simulink model "xNeuralSim_601"  (R2012b)
settings: Solver=FixedStepDiscrete  StartTime=0  StopTime=Inf  FixedStep=.0005  RelTol=1e-3
values from neighbouring files (symbols this model uses):
  cbhwlib_ver_major = 3    [buildXNeuralSim.m]    (also in xNeuralSim_Init.m)
  cbhwlib_ver_minor = 10    [buildXNeuralSim.m]    (also in xNeuralSim_Init.m = 9)
  enableNeuralSim = 1    [xNeuralSim_Init.m]
  max_num_cbpkts = 5    [xNeuralSim_Init.m]
  nch = 192    [xNeuralSim_Init.m]
  nsp_recv_port = 1001    [xNeuralSim_Init.m]
  nsp_send_port = 1002    [xNeuralSim_Init.m]
  sampleSendEnable_NSP1 = 1    [xNeuralSim_Init.m]
  sampleSendEnable_NSP2 = 1    [xNeuralSim_Init.m]
  spikeSendEnable_NSP1 = 1    [xNeuralSim_Init.m]
  spikeSendEnable_NSP2 = 1    [xNeuralSim_Init.m]
  unitMap = unitMap./repmat(sqrt(sum(unitMap.^2)), dimensions, 1)    [xNeuralSim_Init.m]
undefined symbols (not defined in the file or in its folder): macaddr
undefined symbols (not defined in the file): nsp1_pci_bus, nsp1_pci_slot
libraries: xpcethernetlib x15, xpcrtudplib x8, dspmtrx3 x7, xpclib x6, simulink x4, dspsrcs4 x2, xpciplib x2, xpcparallelportlib x1
(part 2 of 2)

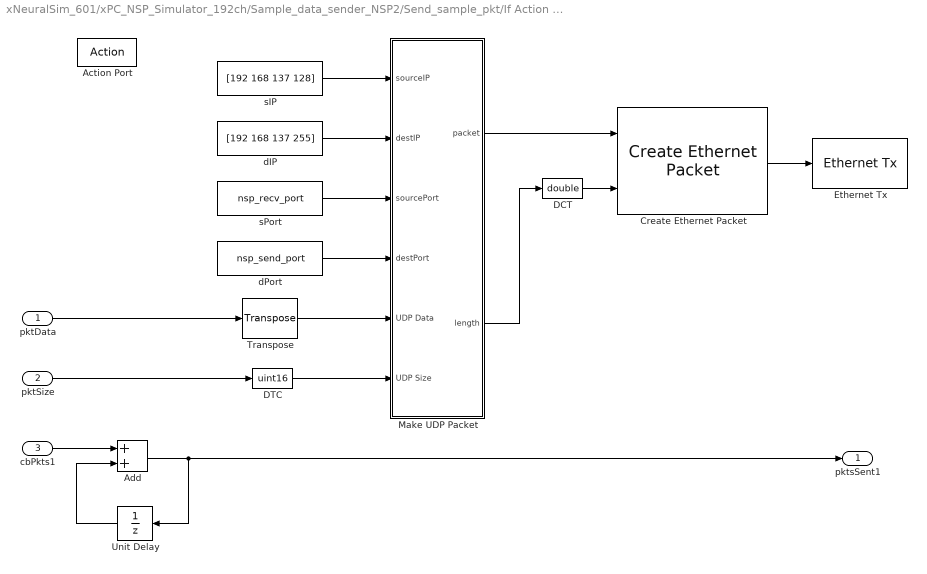
== system xNeuralSim_601/xPC_NSP_Simulator_192ch/Sample_data_sender_NSP2/Send_sample_pkt/If Action Subsystem ==
  pktData : Inport
  pktSize : Inport  Port=2
  cbPkts1 : Inport  Port=3
  Action Port : ActionPort  ActionType=then
  Add : Sum  AccumDataTypeStr=uint32  OutDataTypeStr=uint32
  Create Ethernet Packet : xpcethernetlib/Create Ethernet Packet   DstMac=macaddr('ff:ff:ff:ff:ff:ff')  EtherType=hex2dec('0800')
  DCT : DataTypeConversion  OutDataTypeStr=double
  DTC : DataTypeConversion  OutDataTypeStr=uint16
  Ethernet Tx : xpcethernetlib/Ethernet Tx   ID=2  SampleTime=-1
  Make UDP Packet : Subsystem
  Transpose : dspmtrx3/Transpose  Hermitian=off  overflowFlag=off
  Unit Delay : UnitDelay  SampleTime=-1
  dIP : Constant  Value=[192 168 137 255]  OutDataTypeStr=uint8
  dPort : Constant  Value=nsp_send_port  OutDataTypeStr=uint16
  sIP : Constant  Value=[192 168 137 128]  OutDataTypeStr=uint8
  sPort : Constant  Value=nsp_recv_port  OutDataTypeStr=uint16
  pktsSent1 : Outport  InitialOutput=0
  wires:
  Add/1 -> Unit Delay/1, pktsSent1/1
  Unit Delay/1 -> Add/2
  cbPkts1/1 -> Add/1
  DTC/1 -> Make UDP Packet/6(UDP Size)
  Make UDP Packet/2(length) -> DCT/1
  DCT/1 -> Create Ethernet Packet/2
  Make UDP Packet/1(packet) -> Create Ethernet Packet/1
  sPort/1 -> Make UDP Packet/3(sourcePort)
  Create Ethernet Packet/1 -> Ethernet Tx/1
  sIP/1 -> Make UDP Packet/1(sourceIP)
  dIP/1 -> Make UDP Packet/2(destIP)
  dPort/1 -> Make UDP Packet/4(destPort)
  Transpose/1 -> Make UDP Packet/5(UDP Data)
  pktData/1 -> Transpose/1
  pktSize/1 -> DTC/1

== system xNeuralSim_601/xPC_NSP_Simulator_192ch/Send_config_pkt/If Action Subsystem/Make UDP Packet ==
  note: UDP Data MUST be a uint8 vector of 1472 bytes
      | must pad data with 0s to reach 1472
  sourceIP : Inport
  destIP : Inport  Port=2
  sourcePort : Inport  Port=3
  destPort : Inport  Port=4
  UDP Data : Inport  Port=5
  UDP Size : Inport  Port=6
  Add IP Header : MATLAB Function  TreatAsAtomicUnit=on
  Add UDP Header : MATLAB Function  TreatAsAtomicUnit=on
  packet : Outport
  length : Outport  Port=2
  wires:
  UDP Size/1 -> Add UDP Header/6(UDP_size)
  Add IP Header/2(length) -> length/1
  Add IP Header/1(packet) -> packet/1
  UDP Data/1 -> Add UDP Header/5(UDP_data)
  destPort/1 -> Add UDP Header/4(destPort)
  sourcePort/1 -> Add UDP Header/3(sourcePort)
  destIP/1 -> Add IP Header/2(destIP), Add UDP Header/2(destIP)
  sourceIP/1 -> Add IP Header/1(sourceIP), Add UDP Header/1(sourceIP)
  Add UDP Header/1(packet) -> Add IP Header/3(IP_data)
  Add UDP Header/2(length) -> Add IP Header/4(IP_size)

== system xNeuralSim_601/xPC_NSP_Simulator_192ch/Send_heartbeat/If Action Subsystem/Make UDP Packet ==
  note: UDP Data MUST be a uint8 vector of 1472 bytes
      | must pad data with 0s to reach 1472
  sourceIP : Inport
  destIP : Inport  Port=2
  sourcePort : Inport  Port=3
  destPort : Inport  Port=4
  UDP Data : Inport  Port=5
  UDP Size : Inport  Port=6
  Add IP Header : MATLAB Function  TreatAsAtomicUnit=on
  Add UDP Header : MATLAB Function  TreatAsAtomicUnit=on
  packet : Outport
  length : Outport  Port=2
  wires:
  UDP Size/1 -> Add UDP Header/6(UDP_size)
  Add IP Header/2(length) -> length/1
  Add IP Header/1(packet) -> packet/1
  UDP Data/1 -> Add UDP Header/5(UDP_data)
  destPort/1 -> Add UDP Header/4(destPort)
  sourcePort/1 -> Add UDP Header/3(sourcePort)
  destIP/1 -> Add IP Header/2(destIP), Add UDP Header/2(destIP)
  sourceIP/1 -> Add IP Header/1(sourceIP), Add UDP Header/1(sourceIP)
  Add UDP Header/1(packet) -> Add IP Header/3(IP_data)
  Add UDP Header/2(length) -> Add IP Header/4(IP_size)

== system xNeuralSim_601/xPC_NSP_Simulator_192ch/Send_protocol_pkt/If Action Subsystem/Make UDP Packet ==
  note: UDP Data MUST be a uint8 vector of 1472 bytes
      | must pad data with 0s to reach 1472
  sourceIP : Inport
  destIP : Inport  Port=2
  sourcePort : Inport  Port=3
  destPort : Inport  Port=4
  UDP Data : Inport  Port=5
  UDP Size : Inport  Port=6
  Add IP Header : MATLAB Function  TreatAsAtomicUnit=on
  Add UDP Header : MATLAB Function  TreatAsAtomicUnit=on
  packet : Outport
  length : Outport  Port=2
  wires:
  UDP Size/1 -> Add UDP Header/6(UDP_size)
  Add IP Header/2(length) -> length/1
  Add IP Header/1(packet) -> packet/1
  UDP Data/1 -> Add UDP Header/5(UDP_data)
  destPort/1 -> Add UDP Header/4(destPort)
  sourcePort/1 -> Add UDP Header/3(sourcePort)
  destIP/1 -> Add IP Header/2(destIP), Add UDP Header/2(destIP)
  sourceIP/1 -> Add IP Header/1(sourceIP), Add UDP Header/1(sourceIP)
  Add UDP Header/1(packet) -> Add IP Header/3(IP_data)
  Add UDP Header/2(length) -> Add IP Header/4(IP_size)

== system xNeuralSim_601/xPC_NSP_Simulator_192ch/Send_response_pkt/If Action Subsystem/Make UDP Packet ==
  note: UDP Data MUST be a uint8 vector of 1472 bytes
      | must pad data with 0s to reach 1472
  sourceIP : Inport
  destIP : Inport  Port=2
  sourcePort : Inport  Port=3
  destPort : Inport  Port=4
  UDP Data : Inport  Port=5
  UDP Size : Inport  Port=6
  Add IP Header : MATLAB Function  TreatAsAtomicUnit=on
  Add UDP Header : MATLAB Function  TreatAsAtomicUnit=on
  packet : Outport
  length : Outport  Port=2
  wires:
  UDP Size/1 -> Add UDP Header/6(UDP_size)
  Add IP Header/2(length) -> length/1
  Add IP Header/1(packet) -> packet/1
  UDP Data/1 -> Add UDP Header/5(UDP_data)
  destPort/1 -> Add UDP Header/4(destPort)
  sourcePort/1 -> Add UDP Header/3(sourcePort)
  destIP/1 -> Add IP Header/2(destIP), Add UDP Header/2(destIP)
  sourceIP/1 -> Add IP Header/1(sourceIP), Add UDP Header/1(sourceIP)
  Add UDP Header/1(packet) -> Add IP Header/3(IP_data)
  Add UDP Header/2(length) -> Add IP Header/4(IP_size)

== system xNeuralSim_601/xPC_NSP_Simulator_192ch/Send_runlevel_pkt/If Action Subsystem/Make UDP Packet ==
  note: UDP Data MUST be a uint8 vector of 1472 bytes
      | must pad data with 0s to reach 1472
  sourceIP : Inport
  destIP : Inport  Port=2
  sourcePort : Inport  Port=3
  destPort : Inport  Port=4
  UDP Data : Inport  Port=5
  UDP Size : Inport  Port=6
  Add IP Header : MATLAB Function  TreatAsAtomicUnit=on
  Add UDP Header : MATLAB Function  TreatAsAtomicUnit=on
  packet : Outport
  length : Outport  Port=2
  wires:
  UDP Size/1 -> Add UDP Header/6(UDP_size)
  Add IP Header/2(length) -> length/1
  Add IP Header/1(packet) -> packet/1
  UDP Data/1 -> Add UDP Header/5(UDP_data)
  destPort/1 -> Add UDP Header/4(destPort)
  sourcePort/1 -> Add UDP Header/3(sourcePort)
  destIP/1 -> Add IP Header/2(destIP), Add UDP Header/2(destIP)
  sourceIP/1 -> Add IP Header/1(sourceIP), Add UDP Header/1(sourceIP)
  Add UDP Header/1(packet) -> Add IP Header/3(IP_data)
  Add UDP Header/2(length) -> Add IP Header/4(IP_size)

== system xNeuralSim_601/xPC_NSP_Simulator_192ch/Spike_data_sender_NSP1/Send_sample_pkt/If Action Subsystem ==
  pktData : Inport
  pktSize : Inport  Port=2
  cbPkts : Inport  Port=3
  Action Port : ActionPort  ActionType=then
  Add : Sum  AccumDataTypeStr=uint32  OutDataTypeStr=uint32
  Send_port_1002 : Subsystem  mask(send){Send1=192.168.137.255, Send2=nsp_send_port, Send3=nsp_recv_port, Send4=-1}
      mask prompts: Send1 "IP address to send to (255.255.255.255 for broadcast):"; Send2 "Remote IP port to send to:"; Send3 "Use the following local IP port (-1 for automatic assignment):"; Send4 "Sample time:"
      mask init:
      | Send1 = ipaddr(Send1);
      mask Help: helpview(fullfile(docroot, 'mapfiles', 'xpc.map'), 'RT_UDP_SEND')
      mask Display: disp('UDP\nSend')
  Unit Delay : UnitDelay  SampleTime=-1
  pktsSent : Outport  InitialOutput=0
  wires:
  Add/1 -> Unit Delay/1, pktsSent/1
  Unit Delay/1 -> Add/2
  cbPkts/1 -> Add/1
  pktData/1 -> Send_port_1002/1(In1)
  pktSize/1 -> Send_port_1002/2(In2)

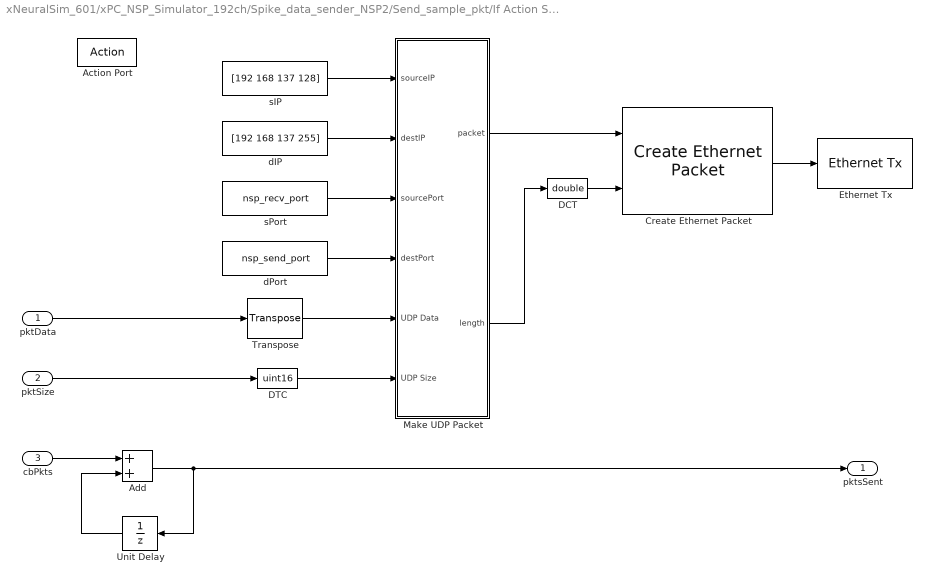
== system xNeuralSim_601/xPC_NSP_Simulator_192ch/Spike_data_sender_NSP2/Send_sample_pkt/If Action Subsystem ==
  pktData : Inport
  pktSize : Inport  Port=2
  cbPkts : Inport  Port=3
  Action Port : ActionPort  ActionType=then
  Add : Sum  AccumDataTypeStr=uint32  OutDataTypeStr=uint32
  Create Ethernet Packet : xpcethernetlib/Create Ethernet Packet   DstMac=macaddr('ff:ff:ff:ff:ff:ff')  EtherType=hex2dec('0800')
  DCT : DataTypeConversion  OutDataTypeStr=double
  DTC : DataTypeConversion  OutDataTypeStr=uint16
  Ethernet Tx : xpcethernetlib/Ethernet Tx   ID=2  SampleTime=-1
  Make UDP Packet : Subsystem
  Transpose : dspmtrx3/Transpose  Hermitian=off  overflowFlag=off
  Unit Delay : UnitDelay  SampleTime=-1
  dIP : Constant  Value=[192 168 137 255]  OutDataTypeStr=uint8
  dPort : Constant  Value=nsp_send_port  OutDataTypeStr=uint16
  sIP : Constant  Value=[192 168 137 128]  OutDataTypeStr=uint8
  sPort : Constant  Value=nsp_recv_port  OutDataTypeStr=uint16
  pktsSent : Outport  InitialOutput=0
  wires:
  Add/1 -> Unit Delay/1, pktsSent/1
  Unit Delay/1 -> Add/2
  cbPkts/1 -> Add/1
  DTC/1 -> Make UDP Packet/6(UDP Size)
  Make UDP Packet/2(length) -> DCT/1
  DCT/1 -> Create Ethernet Packet/2
  Make UDP Packet/1(packet) -> Create Ethernet Packet/1
  sPort/1 -> Make UDP Packet/3(sourcePort)
  Create Ethernet Packet/1 -> Ethernet Tx/1
  sIP/1 -> Make UDP Packet/1(sourceIP)
  dIP/1 -> Make UDP Packet/2(destIP)
  dPort/1 -> Make UDP Packet/4(destPort)
  Transpose/1 -> Make UDP Packet/5(UDP Data)
  pktData/1 -> Transpose/1
  pktSize/1 -> DTC/1

== system xNeuralSim_601/xPC_NSP_Simulator_192ch/Sample_data_sender_NSP1/Send_sample_pkt/If Action Subsystem/Send_port_1002 ==
  In1 : Inport  OutDataTypeStr=uint8
  In2 : Inport  Port=2  OutDataTypeStr=double
  "Compose " : S-Function  FunctionName=xpcnbcompose  EnableBusSupport=off  mask(xpcnbcompose){}
      mask help: Network Buffer Compose
      mask init:
      | mxpcnbcompose(2);
      mask Help: helpview(fullfile(docroot, 'mapfiles', 'xpc.map'), 'NB_Compose')
      mask Display: disp('NB Compose\n');port_label('input', 2, 'length');
  "UDP Produce " : S-Function  Priority=5  FunctionName=xpcudpproduce  Parameters=Group, SrcIp, sip, DstIp, dip, LocPort, lup, RemPort, rup, SampleTime  EnableBusSupport=off  mask(udpproduce){Group=0, sip=Auto, SrcIp=0.0.0.0, dip=Specify, DstIp=Send1, rup=Specify, RemPort=Send2, lup=Auto, LocPort=Send3, SampleTime=Send4}
      mask prompts: Group "IP Group"; sip "Source IP Address"; SrcIp "Source IP Address"; dip "Destination IP Address"; DstIp "IP address to send to (255.255.255.255 for broadcast):"; rup "Remote UDP Port"; RemPort "Remote IP port to send to:"; lup "Local UDP Port"; LocPort "Use the following local IP port (-1 for automatic assignment):"; SampleTime "Sample time:"
      mask help: UDP Produce
      mask init:
      | if LocPort == -1
      |     lup = 3;
      | else
      |     lup = 1;
      | end
      | 
      | SrcIp = ipaddr(SrcIp);
      | DstIp = ipaddr(DstIp);
      mask Help: helpview(fullfile(docroot, 'mapfiles', 'xpc.map'), 'RT_UDP_PRODUCE')
      mask TypeOptions sip: Specify | Port | Auto
      mask TypeOptions dip: Specify | Port
      mask TypeOptions rup: Specify | Port
      mask TypeOptions lup: Specify | Port | Auto
      mask Display: disp('UDP Produce');
  "UDP Tx " : xpciplib/UDP Tx   Priority=5  Group=0  TTL=-1  ToS=-1  SampleTime=Send4
  wires:
  "UDP Produce "/1 -> "UDP Tx "/1
  "Compose "/1 -> "UDP Produce "/1
  In1/1 -> "Compose "/1
  In2/1 -> "Compose "/2

== system xNeuralSim_601/xPC_NSP_Simulator_192ch/Sample_data_sender_NSP2/Send_sample_pkt/If Action Subsystem/Make UDP Packet ==
  note: UDP Data MUST be a uint8 vector of 1472 bytes
      | must pad data with 0s to reach 1472
  sourceIP : Inport
  destIP : Inport  Port=2
  sourcePort : Inport  Port=3
  destPort : Inport  Port=4
  UDP Data : Inport  Port=5
  UDP Size : Inport  Port=6
  Add IP Header : MATLAB Function  TreatAsAtomicUnit=on
  Add UDP Header : MATLAB Function  TreatAsAtomicUnit=on
  packet : Outport
  length : Outport  Port=2
  wires:
  UDP Size/1 -> Add UDP Header/6(UDP_size)
  Add IP Header/2(length) -> length/1
  Add IP Header/1(packet) -> packet/1
  UDP Data/1 -> Add UDP Header/5(UDP_data)
  destPort/1 -> Add UDP Header/4(destPort)
  sourcePort/1 -> Add UDP Header/3(sourcePort)
  destIP/1 -> Add IP Header/2(destIP), Add UDP Header/2(destIP)
  sourceIP/1 -> Add IP Header/1(sourceIP), Add UDP Header/1(sourceIP)
  Add UDP Header/1(packet) -> Add IP Header/3(IP_data)
  Add UDP Header/2(length) -> Add IP Header/4(IP_size)

== system xNeuralSim_601/xPC_NSP_Simulator_192ch/Spike_data_sender_NSP1/Send_sample_pkt/If Action Subsystem/Send_port_1002 ==
  In1 : Inport  OutDataTypeStr=uint8
  In2 : Inport  Port=2  OutDataTypeStr=double
  "Compose " : S-Function  FunctionName=xpcnbcompose  EnableBusSupport=off  mask(xpcnbcompose){}
      mask help: Network Buffer Compose
      mask init:
      | mxpcnbcompose(2);
      mask Help: helpview(fullfile(docroot, 'mapfiles', 'xpc.map'), 'NB_Compose')
      mask Display: disp('NB Compose\n');port_label('input', 2, 'length');
  "UDP Produce " : S-Function  Priority=5  FunctionName=xpcudpproduce  Parameters=Group, SrcIp, sip, DstIp, dip, LocPort, lup, RemPort, rup, SampleTime  EnableBusSupport=off  mask(udpproduce){Group=0, sip=Auto, SrcIp=0.0.0.0, dip=Specify, DstIp=Send1, rup=Specify, RemPort=Send2, lup=Auto, LocPort=Send3, SampleTime=Send4}
      mask prompts: Group "IP Group"; sip "Source IP Address"; SrcIp "Source IP Address"; dip "Destination IP Address"; DstIp "IP address to send to (255.255.255.255 for broadcast):"; rup "Remote UDP Port"; RemPort "Remote IP port to send to:"; lup "Local UDP Port"; LocPort "Use the following local IP port (-1 for automatic assignment):"; SampleTime "Sample time:"
      mask help: UDP Produce
      mask init:
      | if LocPort == -1
      |     lup = 3;
      | else
      |     lup = 1;
      | end
      | 
      | SrcIp = ipaddr(SrcIp);
      | DstIp = ipaddr(DstIp);
      mask Help: helpview(fullfile(docroot, 'mapfiles', 'xpc.map'), 'RT_UDP_PRODUCE')
      mask TypeOptions sip: Specify | Port | Auto
      mask TypeOptions dip: Specify | Port
      mask TypeOptions rup: Specify | Port
      mask TypeOptions lup: Specify | Port | Auto
      mask Display: disp('UDP Produce');
  "UDP Tx " : xpciplib/UDP Tx   Priority=5  Group=0  TTL=-1  ToS=-1  SampleTime=Send4
  wires:
  "UDP Produce "/1 -> "UDP Tx "/1
  "Compose "/1 -> "UDP Produce "/1
  In1/1 -> "Compose "/1
  In2/1 -> "Compose "/2

== system xNeuralSim_601/xPC_NSP_Simulator_192ch/Spike_data_sender_NSP2/Send_sample_pkt/If Action Subsystem/Make UDP Packet ==
  note: UDP Data MUST be a uint8 vector of 1472 bytes
      | must pad data with 0s to reach 1472
  sourceIP : Inport
  destIP : Inport  Port=2
  sourcePort : Inport  Port=3
  destPort : Inport  Port=4
  UDP Data : Inport  Port=5
  UDP Size : Inport  Port=6
  Add IP Header : MATLAB Function  TreatAsAtomicUnit=on
  Add UDP Header : MATLAB Function  TreatAsAtomicUnit=on
  packet : Outport
  length : Outport  Port=2
  wires:
  UDP Size/1 -> Add UDP Header/6(UDP_size)
  Add IP Header/2(length) -> length/1
  Add IP Header/1(packet) -> packet/1
  UDP Data/1 -> Add UDP Header/5(UDP_data)
  destPort/1 -> Add UDP Header/4(destPort)
  sourcePort/1 -> Add UDP Header/3(sourcePort)
  destIP/1 -> Add IP Header/2(destIP), Add UDP Header/2(destIP)
  sourceIP/1 -> Add IP Header/1(sourceIP), Add UDP Header/1(sourceIP)
  Add UDP Header/1(packet) -> Add IP Header/3(IP_data)
  Add UDP Header/2(length) -> Add IP Header/4(IP_size)

== matlab function xNeuralSim_601/xPC_NSP_Simulator_192ch/Send_heartbeat/If Action Subsystem/Make UDP Packet/Add IP Header ==
  data: sourceIP input uint8 size=[1 4]; packet output uint8; destIP input uint8 size=[1 4]; IP_data input uint8; IP_size input uint16 size=[1 1]; length output uint16 size=[1 1]
function [packet, length] = makeIP(sourceIP, destIP, IP_data, IP_size)
% create IP packet

FFFF = uint16(hex2dec('FFFF'));

version_IHL = uint8(69); % IPv4 and IP header length of 5
ToS = uint8(0); % no QOS on network

length = IP_size + uint16(20); % hardcode header length to 5

length_BE = (typecast(length, 'uint8')); % change to big endian
length_BE = length_BE(end:-1:1);

% counter
persistent ID % identification
if isempty(ID)
    ID = uint16(0);
else
    ID = ID + 1;
end

ff = [ uint8(bin2dec('01000000')) 0 ]; % don't fragment packets

TTL = uint8(10); % ttl to 10 seconds/hops

protocol = uint8(hex2dec('11')); % UDP Protocol


header = [ version_IHL ToS length_BE typecast(ID, 'uint8') ff TTL protocol 0 0 sourceIP destIP];

% header(11:12) = typecast(bitcmp(uint16(sum( typecast(bitcmp(header), 'uint16') ))), 'uint8'); % checksum

checksum = FFFF - uint16(mod( uint32(sum( typecast(header, 'uint16') )), uint32(FFFF) ));
header(11:12) = typecast(checksum, 'uint8');

packet = [ header IP_data ];

== matlab function xNeuralSim_601/NeuralSim/MATLAB Function ==
  data: sampleData output; numSamples output; spikeCounts output; numSpikes output; velPacket input; unitMap input; spikeRates output; noise input
function [sampleData,numSamples,spikeCounts,numSpikes,spikeRates]  = fcn(velPacket,unitMap,noise)
%#codegen
persistent t lfp lfpAmpScale scaleTolerance;

if isempty(scaleTolerance)
    scaleTolerance = 1;
end

ch=192;
sigLen = 15;
sampFreq = 30000;

velPacket(4) = velPacket(4) - .5; % rescale the click
%CP, 2015-01-19
%velPacket(4) = velPacket(4)*3;

cursorMap = unitMap'-repmat([velPacket]',[ch 1]);

rho=sqrt(cursorMap(:,1).^2+cursorMap(:,2).^2 + cursorMap(:,3).^2+cursorMap(:,4).^2)-.6;

% Xa=(cursorMap(:,1))./(cursorMap(:,2)+10^-10);

% ArcTan can be computed via a Taylor Approximation (for speed)
% theta=Xa-1/3*Xa.^3+1/5*Xa.^5-1/7*Xa.^7+1/9*Xa.^9+1/11*Xa.^11;

% CosTheta=1-1/2*theta.^2+1/24*theta.^4-1/120*theta.^6;
% CosTheta = zeros(size(rho));

randTolerance = .1;


SpikeRateSec = (20 * (rho)); %.*(CosTheta+1);
SpikeRateSec = SpikeRateSec * scaleTolerance;
lfpAmpMod = 5 + 45 * max(rho,0); %.*(CosTheta+1);
lfpAmpMod = lfpAmpMod * scaleTolerance;
lfpAmpScaleBase = 50;


% Spikes

spikeProb = repmat(SpikeRateSec * sigLen / sampFreq,[1 sigLen]);

probMatrix = (rand(ch,sigLen) > (1-spikeProb));

spikes = zeros(size(probMatrix));

spikeCounter = sum(probMatrix,2);

totalNumSpikes = sum(spikeCounter);

spikes(probMatrix) =  -80;



fbands=[5 10 20 40 80 160 320];
% fbands=[5];

% sigLen=samples;


maxLen=sigLen*400; % must enforce maxLen as 2N multiple of sigLen

% t = []; lfp = [];
if isempty(t)
    t=0;
    lfp=zeros(ch,maxLen,length(fbands));
    lfpAmpScale = lfpAmpScaleBase*ones(ch,1).* (lfpAmpMod);
    for f=1:length(fbands)
        lfp(:,1:maxLen,f)=((1/f*(sin(2*pi*(1/sampFreq)*((fbands(f)))*repmat([1:maxLen],[ch 1 1])+repmat(rand(ch,1)*2*pi,[1 maxLen 1])))));
    end
end


data = int16((mean(lfp(:,t+1:t+sigLen,:) .* repmat(lfpAmpScale,[1 sigLen length(fbands)]),3)));

% Prep for next iteration

t=t+sigLen;
%a=round(mod(t+1,slen/plen)*plen);

if t + sigLen == maxLen/2
    lfpAmpScale = lfpAmpScaleBase*ones(ch,1) .* (lfpAmpMod);
end

if t + sigLen == maxLen
    t=0;
    lfpAmpScale = lfpAmpScaleBase*ones(ch,1) .* (lfpAmpMod);
    scaleTolerance = rand(1) * randTolerance * 2 + (1-randTolerance);
end


% Collect outputs

sampleData = data+noise+int16(spikes);
numSamples = int32(sigLen);

spikeCounts = int32(spikeCounter);
numSpikes = totalNumSpikes;
spikeRates = [SpikeRateSec; zeros(ch*2,1)];

% to=t;

end

== matlab function xNeuralSim_601/xPC_NSP_Simulator_192ch/Send_heartbeat/If Action Subsystem/Make UDP Packet/Add UDP Header ==
  data: sourceIP input uint8 size=[1 4]; packet output; destIP input uint8 size=[1 4]; sourcePort input uint16 size=[1 1]; destPort input uint16 size=[1 1]; UDP_data input uint8; UDP_size input uint16 size=[1 1]; length output uint16 size=[1 1]
function [packet, length] = makeUDP(sourceIP, destIP, sourcePort, destPort, UDP_data, UDP_size)
% create UDP packet

% sourceIP and destIP are 1x4 uint8 of the IP (in address order)
% sourcePort and destPort are uint16
% UDP_data is uint8 of 1xN packet data
% UDP_size is uint16 size of UDP_data
%
% NOTE: UDP_size MUST BE EVEN
FFFF = uint16(hex2dec('FFFF'));

protocol = uint8(hex2dec('11'));

length = UDP_size + uint16(8);

length_BE = (typecast(length, 'uint8')); % flip to big endian
length_BE = length_BE(end:-1:1);

sourcePort_BE = (typecast(sourcePort, 'uint8'));
sourcePort_BE = sourcePort_BE(end:-1:1);

destPort_BE   = (typecast(destPort,   'uint8'));
destPort_BE = destPort_BE(end:-1:1);

header = [sourcePort_BE destPort_BE length_BE uint8([0 0])];

pseudoHeader = [sourceIP destIP uint8(0) protocol length_BE];

% header(7:8) = typecast( bitcmp(uint16(sum( typecast(bitcmp([pseudoHeader header UDP_data]), 'uint16') ))), 'uint8');


checksum = FFFF - uint16(mod( uint32(sum( typecast([pseudoHeader header UDP_data], 'uint16') )), uint32(FFFF) ));
header(7:8) = typecast(checksum, 'uint8');

packet = [ header UDP_data ];

== matlab function xNeuralSim_601/xPC_NSP_Simulator_192ch/Send_config_pkt/If Action Subsystem/Make UDP Packet/Add IP Header ==
  data: sourceIP input uint8 size=[1 4]; packet output uint8; destIP input uint8 size=[1 4]; IP_data input uint8; IP_size input uint16 size=[1 1]; length output uint16 size=[1 1]
function [packet, length] = makeIP(sourceIP, destIP, IP_data, IP_size)
% create IP packet

FFFF = uint16(hex2dec('FFFF'));

version_IHL = uint8(69); % IPv4 and IP header length of 5
ToS = uint8(0); % no QOS on network

length = IP_size + uint16(20); % hardcode header length to 5

length_BE = (typecast(length, 'uint8')); % change to big endian
length_BE = length_BE(end:-1:1);

% counter
persistent ID % identification
if isempty(ID)
    ID = uint16(0);
else
    ID = ID + 1;
end

ff = [ uint8(bin2dec('01000000')) 0 ]; % don't fragment packets

TTL = uint8(10); % ttl to 10 seconds/hops

protocol = uint8(hex2dec('11')); % UDP Protocol


header = [ version_IHL ToS length_BE typecast(ID, 'uint8') ff TTL protocol 0 0 sourceIP destIP];

% header(11:12) = typecast(bitcmp(uint16(sum( typecast(bitcmp(header), 'uint16') ))), 'uint8'); % checksum

checksum = FFFF - uint16(mod( uint32(sum( typecast(header, 'uint16') )), uint32(FFFF) ));
header(11:12) = typecast(checksum, 'uint8');

packet = [ header IP_data ];

== matlab function xNeuralSim_601/xPC_NSP_Simulator_192ch/Send_config_pkt/If Action Subsystem/Make UDP Packet/Add UDP Header ==
  data: sourceIP input uint8 size=[1 4]; packet output; destIP input uint8 size=[1 4]; sourcePort input uint16 size=[1 1]; destPort input uint16 size=[1 1]; UDP_data input uint8; UDP_size input uint16 size=[1 1]; length output uint16 size=[1 1]
function [packet, length] = makeUDP(sourceIP, destIP, sourcePort, destPort, UDP_data, UDP_size)
% create UDP packet

% sourceIP and destIP are 1x4 uint8 of the IP (in address order)
% sourcePort and destPort are uint16
% UDP_data is uint8 of 1xN packet data
% UDP_size is uint16 size of UDP_data
%
% NOTE: UDP_size MUST BE EVEN
FFFF = uint16(hex2dec('FFFF'));

protocol = uint8(hex2dec('11'));

length = UDP_size + uint16(8);

length_BE = (typecast(length, 'uint8')); % flip to big endian
length_BE = length_BE(end:-1:1);

sourcePort_BE = (typecast(sourcePort, 'uint8'));
sourcePort_BE = sourcePort_BE(end:-1:1);

destPort_BE   = (typecast(destPort,   'uint8'));
destPort_BE = destPort_BE(end:-1:1);

header = [sourcePort_BE destPort_BE length_BE uint8([0 0])];

pseudoHeader = [sourceIP destIP uint8(0) protocol length_BE];

% header(7:8) = typecast( bitcmp(uint16(sum( typecast(bitcmp([pseudoHeader header UDP_data]), 'uint16') ))), 'uint8');


checksum = FFFF - uint16(mod( uint32(sum( typecast([pseudoHeader header UDP_data], 'uint16') )), uint32(FFFF) ));
header(7:8) = typecast(checksum, 'uint8');

packet = [ header UDP_data ];

== matlab function xNeuralSim_601/xPC_NSP_Simulator_192ch/Send_response_pkt/If Action Subsystem/Make UDP Packet/Add IP Header ==
  data: sourceIP input uint8 size=[1 4]; packet output uint8; destIP input uint8 size=[1 4]; IP_data input uint8; IP_size input uint16 size=[1 1]; length output uint16 size=[1 1]
function [packet, length] = makeIP(sourceIP, destIP, IP_data, IP_size)
% create IP packet

FFFF = uint16(hex2dec('FFFF'));

version_IHL = uint8(69); % IPv4 and IP header length of 5
ToS = uint8(0); % no QOS on network

length = IP_size + uint16(20); % hardcode header length to 5

length_BE = (typecast(length, 'uint8')); % change to big endian
length_BE = length_BE(end:-1:1);

% counter
persistent ID % identification
if isempty(ID)
    ID = uint16(0);
else
    ID = ID + 1;
end

ff = [ uint8(bin2dec('01000000')) 0 ]; % don't fragment packets

TTL = uint8(10); % ttl to 10 seconds/hops

protocol = uint8(hex2dec('11')); % UDP Protocol


header = [ version_IHL ToS length_BE typecast(ID, 'uint8') ff TTL protocol 0 0 sourceIP destIP];

% header(11:12) = typecast(bitcmp(uint16(sum( typecast(bitcmp(header), 'uint16') ))), 'uint8'); % checksum

checksum = FFFF - uint16(mod( uint32(sum( typecast(header, 'uint16') )), uint32(FFFF) ));
header(11:12) = typecast(checksum, 'uint8');

packet = [ header IP_data ];

== matlab function xNeuralSim_601/xPC_NSP_Simulator_192ch/Send_response_pkt/If Action Subsystem/Make UDP Packet/Add UDP Header ==
  data: sourceIP input uint8 size=[1 4]; packet output; destIP input uint8 size=[1 4]; sourcePort input uint16 size=[1 1]; destPort input uint16 size=[1 1]; UDP_data input uint8; UDP_size input uint16 size=[1 1]; length output uint16 size=[1 1]
function [packet, length] = makeUDP(sourceIP, destIP, sourcePort, destPort, UDP_data, UDP_size)
% create UDP packet

% sourceIP and destIP are 1x4 uint8 of the IP (in address order)
% sourcePort and destPort are uint16
% UDP_data is uint8 of 1xN packet data
% UDP_size is uint16 size of UDP_data
%
% NOTE: UDP_size MUST BE EVEN
FFFF = uint16(hex2dec('FFFF'));

protocol = uint8(hex2dec('11'));

length = UDP_size + uint16(8);

length_BE = (typecast(length, 'uint8')); % flip to big endian
length_BE = length_BE(end:-1:1);

sourcePort_BE = (typecast(sourcePort, 'uint8'));
sourcePort_BE = sourcePort_BE(end:-1:1);

destPort_BE   = (typecast(destPort,   'uint8'));
destPort_BE = destPort_BE(end:-1:1);

header = [sourcePort_BE destPort_BE length_BE uint8([0 0])];

pseudoHeader = [sourceIP destIP uint8(0) protocol length_BE];

% header(7:8) = typecast( bitcmp(uint16(sum( typecast(bitcmp([pseudoHeader header UDP_data]), 'uint16') ))), 'uint8');


checksum = FFFF - uint16(mod( uint32(sum( typecast([pseudoHeader header UDP_data], 'uint16') )), uint32(FFFF) ));
header(7:8) = typecast(checksum, 'uint8');

packet = [ header UDP_data ];

== matlab function xNeuralSim_601/xPC_NSP_Simulator_192ch/Send_runlevel_pkt/If Action Subsystem/Make UDP Packet/Add IP Header ==
  data: sourceIP input uint8 size=[1 4]; packet output uint8; destIP input uint8 size=[1 4]; IP_data input uint8; IP_size input uint16 size=[1 1]; length output uint16 size=[1 1]
function [packet, length] = makeIP(sourceIP, destIP, IP_data, IP_size)
% create IP packet

FFFF = uint16(hex2dec('FFFF'));

version_IHL = uint8(69); % IPv4 and IP header length of 5
ToS = uint8(0); % no QOS on network

length = IP_size + uint16(20); % hardcode header length to 5

length_BE = (typecast(length, 'uint8')); % change to big endian
length_BE = length_BE(end:-1:1);

% counter
persistent ID % identification
if isempty(ID)
    ID = uint16(0);
else
    ID = ID + 1;
end

ff = [ uint8(bin2dec('01000000')) 0 ]; % don't fragment packets

TTL = uint8(10); % ttl to 10 seconds/hops

protocol = uint8(hex2dec('11')); % UDP Protocol


header = [ version_IHL ToS length_BE typecast(ID, 'uint8') ff TTL protocol 0 0 sourceIP destIP];

% header(11:12) = typecast(bitcmp(uint16(sum( typecast(bitcmp(header), 'uint16') ))), 'uint8'); % checksum

checksum = FFFF - uint16(mod( uint32(sum( typecast(header, 'uint16') )), uint32(FFFF) ));
header(11:12) = typecast(checksum, 'uint8');

packet = [ header IP_data ];

== matlab function xNeuralSim_601/xpcTargetClockGenerator/cerebus Parallel ==
  data: digitalOut output double size=1
function digitalOut = xpcTargetClock()
%#codegen
persistent clockVal

if isempty(clockVal)
    clockVal = uint32([1;0]);
end

clockVal = circshift(clockVal,1);

digitalOut = double( bitget(clockVal(1),  1) ); % which bit of that uint32?

== matlab function xNeuralSim_601/xPC_NSP_Simulator_192ch/Send_runlevel_pkt/If Action Subsystem/Make UDP Packet/Add UDP Header ==
  data: sourceIP input uint8 size=[1 4]; packet output; destIP input uint8 size=[1 4]; sourcePort input uint16 size=[1 1]; destPort input uint16 size=[1 1]; UDP_data input uint8; UDP_size input uint16 size=[1 1]; length output uint16 size=[1 1]
function [packet, length] = makeUDP(sourceIP, destIP, sourcePort, destPort, UDP_data, UDP_size)
% create UDP packet

% sourceIP and destIP are 1x4 uint8 of the IP (in address order)
% sourcePort and destPort are uint16
% UDP_data is uint8 of 1xN packet data
% UDP_size is uint16 size of UDP_data
%
% NOTE: UDP_size MUST BE EVEN
FFFF = uint16(hex2dec('FFFF'));

protocol = uint8(hex2dec('11'));

length = UDP_size + uint16(8);

length_BE = (typecast(length, 'uint8')); % flip to big endian
length_BE = length_BE(end:-1:1);

sourcePort_BE = (typecast(sourcePort, 'uint8'));
sourcePort_BE = sourcePort_BE(end:-1:1);

destPort_BE   = (typecast(destPort,   'uint8'));
destPort_BE = destPort_BE(end:-1:1);

header = [sourcePort_BE destPort_BE length_BE uint8([0 0])];

pseudoHeader = [sourceIP destIP uint8(0) protocol length_BE];

% header(7:8) = typecast( bitcmp(uint16(sum( typecast(bitcmp([pseudoHeader header UDP_data]), 'uint16') ))), 'uint8');


checksum = FFFF - uint16(mod( uint32(sum( typecast([pseudoHeader header UDP_data], 'uint16') )), uint32(FFFF) ));
header(7:8) = typecast(checksum, 'uint8');

packet = [ header UDP_data ];

== matlab function xNeuralSim_601/xPC_NSP_Simulator_192ch/Send_protocol_pkt/If Action Subsystem/Make UDP Packet/Add IP Header ==
  data: sourceIP input uint8 size=[1 4]; packet output uint8; destIP input uint8 size=[1 4]; IP_data input uint8; IP_size input uint16 size=[1 1]; length output uint16 size=[1 1]
function [packet, length] = makeIP(sourceIP, destIP, IP_data, IP_size)
% create IP packet

FFFF = uint16(hex2dec('FFFF'));

version_IHL = uint8(69); % IPv4 and IP header length of 5
ToS = uint8(0); % no QOS on network

length = IP_size + uint16(20); % hardcode header length to 5

length_BE = (typecast(length, 'uint8')); % change to big endian
length_BE = length_BE(end:-1:1);

% counter
persistent ID % identification
if isempty(ID)
    ID = uint16(0);
else
    ID = ID + 1;
end

ff = [ uint8(bin2dec('01000000')) 0 ]; % don't fragment packets

TTL = uint8(10); % ttl to 10 seconds/hops

protocol = uint8(hex2dec('11')); % UDP Protocol


header = [ version_IHL ToS length_BE typecast(ID, 'uint8') ff TTL protocol 0 0 sourceIP destIP];

% header(11:12) = typecast(bitcmp(uint16(sum( typecast(bitcmp(header), 'uint16') ))), 'uint8'); % checksum

checksum = FFFF - uint16(mod( uint32(sum( typecast(header, 'uint16') )), uint32(FFFF) ));
header(11:12) = typecast(checksum, 'uint8');

packet = [ header IP_data ];

== matlab function xNeuralSim_601/xPC_NSP_Simulator_192ch/Send_protocol_pkt/If Action Subsystem/Make UDP Packet/Add UDP Header ==
  data: sourceIP input uint8 size=[1 4]; packet output; destIP input uint8 size=[1 4]; sourcePort input uint16 size=[1 1]; destPort input uint16 size=[1 1]; UDP_data input uint8; UDP_size input uint16 size=[1 1]; length output uint16 size=[1 1]
function [packet, length] = makeUDP(sourceIP, destIP, sourcePort, destPort, UDP_data, UDP_size)
% create UDP packet

% sourceIP and destIP are 1x4 uint8 of the IP (in address order)
% sourcePort and destPort are uint16
% UDP_data is uint8 of 1xN packet data
% UDP_size is uint16 size of UDP_data
%
% NOTE: UDP_size MUST BE EVEN
FFFF = uint16(hex2dec('FFFF'));

protocol = uint8(hex2dec('11'));

length = UDP_size + uint16(8);

length_BE = (typecast(length, 'uint8')); % flip to big endian
length_BE = length_BE(end:-1:1);

sourcePort_BE = (typecast(sourcePort, 'uint8'));
sourcePort_BE = sourcePort_BE(end:-1:1);

destPort_BE   = (typecast(destPort,   'uint8'));
destPort_BE = destPort_BE(end:-1:1);

header = [sourcePort_BE destPort_BE length_BE uint8([0 0])];

pseudoHeader = [sourceIP destIP uint8(0) protocol length_BE];

% header(7:8) = typecast( bitcmp(uint16(sum( typecast(bitcmp([pseudoHeader header UDP_data]), 'uint16') ))), 'uint8');


checksum = FFFF - uint16(mod( uint32(sum( typecast([pseudoHeader header UDP_data], 'uint16') )), uint32(FFFF) ));
header(7:8) = typecast(checksum, 'uint8');

packet = [ header UDP_data ];

== matlab function xNeuralSim_601/xPC_NSP_Simulator_192ch/Sample_data_sender_NSP2/Send_sample_pkt/If Action Subsystem/Make UDP Packet/Add IP Header ==
  data: sourceIP input uint8 size=[1 4]; packet output uint8; destIP input uint8 size=[1 4]; IP_data input uint8; IP_size input uint16 size=[1 1]; length output uint16 size=[1 1]
function [packet, length] = makeIP(sourceIP, destIP, IP_data, IP_size)
% create IP packet

FFFF = uint16(hex2dec('FFFF'));

version_IHL = uint8(69); % IPv4 and IP header length of 5
ToS = uint8(0); % no QOS on network

length = IP_size + uint16(20); % hardcode header length to 5

length_BE = (typecast(length, 'uint8')); % change to big endian
length_BE = length_BE(end:-1:1);

% counter
persistent ID % identification
if isempty(ID)
    ID = uint16(0);
else
    ID = ID + 1;
end

ff = [ uint8(bin2dec('01000000')) 0 ]; % don't fragment packets

TTL = uint8(10); % ttl to 10 seconds/hops

protocol = uint8(hex2dec('11')); % UDP Protocol


header = [ version_IHL ToS length_BE typecast(ID, 'uint8') ff TTL protocol 0 0 sourceIP destIP];

% header(11:12) = typecast(bitcmp(uint16(sum( typecast(bitcmp(header), 'uint16') ))), 'uint8'); % checksum

checksum = FFFF - uint16(mod( uint32(sum( typecast(header, 'uint16') )), uint32(FFFF) ));
header(11:12) = typecast(checksum, 'uint8');

packet = [ header IP_data ];

== matlab function xNeuralSim_601/xPC_NSP_Simulator_192ch/Sample_data_sender_NSP2/Send_sample_pkt/If Action Subsystem/Make UDP Packet/Add UDP Header ==
  data: sourceIP input uint8 size=[1 4]; packet output; destIP input uint8 size=[1 4]; sourcePort input uint16 size=[1 1]; destPort input uint16 size=[1 1]; UDP_data input uint8; UDP_size input uint16 size=[1 1]; length output uint16 size=[1 1]
function [packet, length] = makeUDP(sourceIP, destIP, sourcePort, destPort, UDP_data, UDP_size)
% create UDP packet

% sourceIP and destIP are 1x4 uint8 of the IP (in address order)
% sourcePort and destPort are uint16
% UDP_data is uint8 of 1xN packet data
% UDP_size is uint16 size of UDP_data
%
% NOTE: UDP_size MUST BE EVEN
FFFF = uint16(hex2dec('FFFF'));

protocol = uint8(hex2dec('11'));

length = UDP_size + uint16(8);

length_BE = (typecast(length, 'uint8')); % flip to big endian
length_BE = length_BE(end:-1:1);

sourcePort_BE = (typecast(sourcePort, 'uint8'));
sourcePort_BE = sourcePort_BE(end:-1:1);

destPort_BE   = (typecast(destPort,   'uint8'));
destPort_BE = destPort_BE(end:-1:1);

header = [sourcePort_BE destPort_BE length_BE uint8([0 0])];

pseudoHeader = [sourceIP destIP uint8(0) protocol length_BE];

% header(7:8) = typecast( bitcmp(uint16(sum( typecast(bitcmp([pseudoHeader header UDP_data]), 'uint16') ))), 'uint8');


checksum = FFFF - uint16(mod( uint32(sum( typecast([pseudoHeader header UDP_data], 'uint16') )), uint32(FFFF) ));
header(7:8) = typecast(checksum, 'uint8');

packet = [ header UDP_data ];

== matlab function xNeuralSim_601/xPC_NSP_Simulator_192ch/Spike_data_sender_NSP2/Send_sample_pkt/If Action Subsystem/Make UDP Packet/Add IP Header ==
  data: sourceIP input uint8 size=[1 4]; packet output uint8; destIP input uint8 size=[1 4]; IP_data input uint8; IP_size input uint16 size=[1 1]; length output uint16 size=[1 1]
function [packet, length] = makeIP(sourceIP, destIP, IP_data, IP_size)
% create IP packet

FFFF = uint16(hex2dec('FFFF'));

version_IHL = uint8(69); % IPv4 and IP header length of 5
ToS = uint8(0); % no QOS on network

length = IP_size + uint16(20); % hardcode header length to 5

length_BE = (typecast(length, 'uint8')); % change to big endian
length_BE = length_BE(end:-1:1);

% counter
persistent ID % identification
if isempty(ID)
    ID = uint16(0);
else
    ID = ID + 1;
end

ff = [ uint8(bin2dec('01000000')) 0 ]; % don't fragment packets

TTL = uint8(10); % ttl to 10 seconds/hops

protocol = uint8(hex2dec('11')); % UDP Protocol


header = [ version_IHL ToS length_BE typecast(ID, 'uint8') ff TTL protocol 0 0 sourceIP destIP];

% header(11:12) = typecast(bitcmp(uint16(sum( typecast(bitcmp(header), 'uint16') ))), 'uint8'); % checksum

checksum = FFFF - uint16(mod( uint32(sum( typecast(header, 'uint16') )), uint32(FFFF) ));
header(11:12) = typecast(checksum, 'uint8');

packet = [ header IP_data ];

== matlab function xNeuralSim_601/xPC_NSP_Simulator_192ch/Spike_data_sender_NSP2/Send_sample_pkt/If Action Subsystem/Make UDP Packet/Add UDP Header ==
  data: sourceIP input uint8 size=[1 4]; packet output; destIP input uint8 size=[1 4]; sourcePort input uint16 size=[1 1]; destPort input uint16 size=[1 1]; UDP_data input uint8; UDP_size input uint16 size=[1 1]; length output uint16 size=[1 1]
function [packet, length] = makeUDP(sourceIP, destIP, sourcePort, destPort, UDP_data, UDP_size)
% create UDP packet

% sourceIP and destIP are 1x4 uint8 of the IP (in address order)
% sourcePort and destPort are uint16
% UDP_data is uint8 of 1xN packet data
% UDP_size is uint16 size of UDP_data
%
% NOTE: UDP_size MUST BE EVEN
FFFF = uint16(hex2dec('FFFF'));

protocol = uint8(hex2dec('11'));

length = UDP_size + uint16(8);

length_BE = (typecast(length, 'uint8')); % flip to big endian
length_BE = length_BE(end:-1:1);

sourcePort_BE = (typecast(sourcePort, 'uint8'));
sourcePort_BE = sourcePort_BE(end:-1:1);

destPort_BE   = (typecast(destPort,   'uint8'));
destPort_BE = destPort_BE(end:-1:1);

header = [sourcePort_BE destPort_BE length_BE uint8([0 0])];

pseudoHeader = [sourceIP destIP uint8(0) protocol length_BE];

% header(7:8) = typecast( bitcmp(uint16(sum( typecast(bitcmp([pseudoHeader header UDP_data]), 'uint16') ))), 'uint8');


checksum = FFFF - uint16(mod( uint32(sum( typecast([pseudoHeader header UDP_data], 'uint16') )), uint32(FFFF) ));
header(7:8) = typecast(checksum, 'uint8');

packet = [ header UDP_data ];
